simulink model "fractional_6"  (Simulink 7.4)
settings: Solver=ode45  StartTime=0.0  StopTime=1e-4  FixedStep=.01/(fr*N/M)  MaxStep=1/(3*fr*N)  RelTol=1e-7  AbsTol=1e-3
PreLoadFcn:
  | fr=10e6,fi=99e6,sen=10e6,N=10,M=.015
StartFcn:
  | tic
StopFcn:
  | trun=toc
undefined symbols (not defined in the file or in its folder): dBW, Hz, M, N, One, sen, sided
libraries: powerlib x11, dspstat3 x4, dsparch4 x3, simulink x3, simulink_extras x2, dspsnks4 x2, commsynccomp2 x1
settings Model: Creator=d benson  LastModifiedBy=Dick  ModifiedHistory=digital phase correction added, Benson, Fall 2001  BufferReuse=off
settings DataIOCC: LimitDataPoints=off  SaveOutput=off  SaveTime=off  SignalLoggingName=sigsOut
settings OptimizationCC: BlockReduction=off  BooleanDataType=off  InlineInvariantSignals=on  OptimizeBlockIOStorage=off  BufferReuse=off  ExpressionFolding=off  LocalBlockOutputs=off  InitFltsAndDblsToZero=on
settings DebuggingCC: SaveWithParameterizedLinksMsg=none  SignalResolutionControl=TryResolveAllWithWarning  SolverPrmCheckMsg=none  MultiTaskDSMMsg=warning  MultiTaskCondExecSysMsg=none  StrictBusMsg=None
settings HardwareCC: TargetUnknown=on
settings RTWCC: IncludeERTFirstTime=on
settings GRTTargetCC: TargetFcnLib=ansi_tfl_tmw.mat

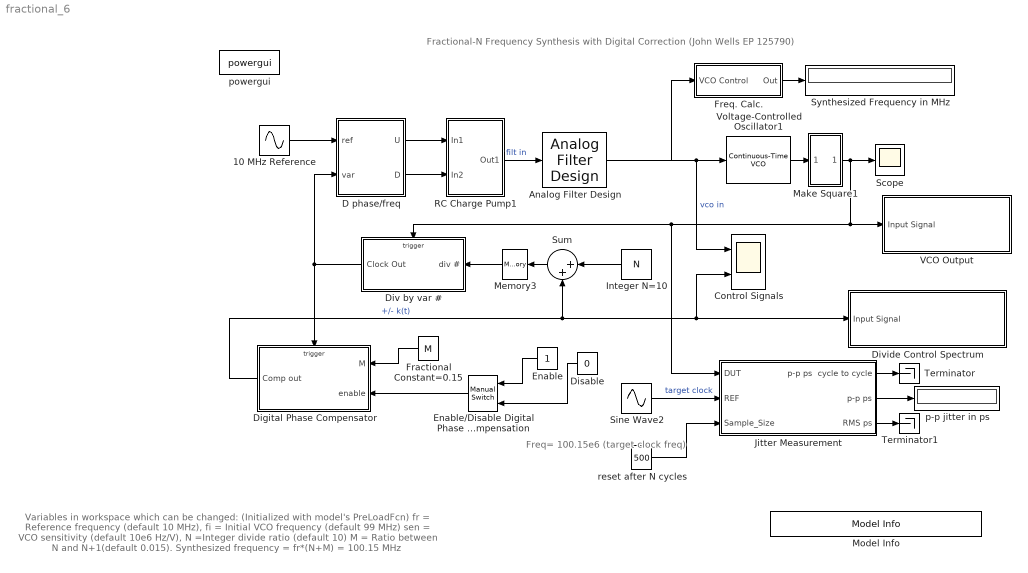
== system fractional_6 ==
  note: Fractional-N Frequency Synthesis with Digital Correction (John Wells EP 125790)
  note: Variables in workspace which can be changed: (Initialized with model's PreLoadFcn)
      | fr = Reference frequency (default 10  MHz),        fi = Initial VCO frequency (default 99 MHz)
      | sen = VCO sensitivity (default 10e6 Hz/V),         N =Integer divide ratio (default 10)
      | M = Ratio between N and N+1(default 0.015).     Synthesized frequency = fr*(N+M) = 100.15 MHz
  note: Freq= 100.15e6 (target clock freq)
  10 MHz Reference : Sin  Amplitude=1  Bias=0  Frequency=2*pi*fr  Phase=0  Samples=10  SampleTime=0  Offset=0
  Analog Filter Design : dsparch4/Analog Filter Design  method=Elliptic  filttype=Lowpass  N=6  Wlo=2*pi*1e6  Whi=80  Rp=2  Rs=80
  Control Signals : Scope  NumInputPorts=2
      settings: TimeRange=0.0001  YMin=0~-7.5  YMax=0.2~7.5  Decimation=51
  "D phase/freq " : Subsystem
  Digital Phase Compensator : Subsystem  TreatAsAtomicUnit=on
  Disable : Constant  Value=0  OutDataType=sfix(16)  OutScaling=2^0
  Div by var # : Subsystem  TreatAsAtomicUnit=on
  Divide Control Spectrum : Subsystem  Description=Spectrum Analyzer  mask{BW=40e6}
      mask prompts: BW "Bandwidth"
      mask Display: fprintf('Baseband Spectrum Analyzer \n  BW=%7.2f MHz', BW/1e6)
  Enable : Constant  OutDataType=sfix(16)  OutScaling=2^0
  Enable/Disable Digital Phase Compensation : simulink/Signal Routing/Manual Switch  SystemSampleTime=-1  sw=1  action=0  varsize=off
  Fractional Constant=0.15 : Constant  Value=M  OutDataType=sfix(16)  OutScaling=2^0
  Freq. Calc. : Subsystem
  Integer N=10 : Constant  Value=N  OutDataType=sfix(16)  OutScaling=2^0
  "Jitter Measurement " : Subsystem
  Make Square1 : Subsystem
      mask Type: Make Square
      mask Description:
      | For input +ve values output is 1
      | For input -ve values output is 0
      mask Display: plot(0,0,100,100,[90,70,70,50,50,30,30,10,10],[20,20,40,40,20,20,40,40,20],[90,87,84,80,76,73,70,67,63,60,57,53,50,47,44,40,36,33,30,27,23,20,17,13,10],[70,65,63,62,63,65,70,75,77,78,77,75,70,65,63,62,63,65,70,75,77,78,77,75,70])
  Memory3 : Memory
  Model Info : simulink/Model-Wide Utilities/Model Info  SystemSampleTime=-1  InitialBlockCM=none  BlockCM=none  Frame=on  DisplayStringWithTags=Copywrite 2005-2010 The MathWorks, Inc.  HorizontalTextAlignment=Center  LeftAlignmentValue=0.5  SourceBlockDiagram=fractional_6  TagMaxNumber=20
  RC Charge Pump1 : Subsystem
  Scope : Scope
      settings: TimeRange=9.98502246630055e-009  YMin=-0.1  YMax=1.1
  Sine Wave2 : Sin  Amplitude=1  Bias=0  Frequency=2*pi*(100.15e6)  Phase=pi/2  Samples=10  SampleTime=0  Offset=0
  Sum : Sum  Inputs=|++  OutDataType=sfix(16)  OutScaling=2^0  SaturateOnIntegerOverflow=on  InputSameDT=on  OutDataTypeStr=Inherit: Same as first input
  "Synthesized Frequency in MHz " : Display
      settings: Decimation=401
  Terminator : Terminator
  Terminator1 : Terminator
  VCO Output : Subsystem  Description=Spectrum Analyzer  mask{BW=4e6, Fc=100.15e6}
      mask prompts: BW "Bandwidth"; Fc "Center Freq"
      mask Display: fprintf('Spectrum Analyzer \n Fc=%7.2f MHz \n BW=%7.2f MHz',Fc/1e6,BW/1e6)
  Voltage-Controlled Oscillator1 : commsynccomp2/Continuous-Time VCO  SystemSampleTime=-1  Ac=1  Fc=fi  Kc=sen  Ph=pi/8
  p-p jitter in ps : Display
  powergui : powerlib/powergui  SystemSampleTime=-1  SimulationMode=Continuous  SampleTime=0  frequency=60  SPID=off  DisableSnubberDevices=off  DisableRonSwitches=off  DisableVfSwitches=off  SwTol=0  Interpol=off  frequencyindice=0  echomessages=off  HookPort=off  DisplayEquations=off  FunctionMessages=off  EnableUseOfTLC=off  x0status=blocks  RestoreLinks=warning  Frange=[0:2:500]  Ylog=off  Xlog=on  ShowGrid=off  save=off  variable=ZData  ZoomFFT=on  StartTime=0.0  cycles=1  DisplayStyle=1  fundamental=60  FreqAxis=off  MaxFrequency=1000  frequencyindicesteady=1  RmsSteady=1  display=off  Ts=0  methode=off
  reset after N cycles : Constant  Value=500  VectorParams1D=off  OutDataType=sfix(16)  OutScaling=2^0
  wires:
  Voltage-Controlled Oscillator1/1 -> Make Square1/1(In1)
  Make Square1/1(Out1) -> Scope/1, VCO Output/1(Input Signal), Div by var #/Trigger, "Jitter Measurement "/1(DUT)
  10 MHz Reference/1 -> "D phase/freq "/1(ref)
  Div by var #/1(Clock Out) -> "D phase/freq "/2(var), Digital Phase Compensator/Trigger
  Sum/1 -> Memory3/1
  Integer N=10/1 -> Sum/1
  Freq. Calc./1(Out) -> "Synthesized Frequency in MHz "/1
  Analog Filter Design/1 -> Control Signals/1, Freq. Calc./1(VCO Control), Voltage-Controlled Oscillator1/1  "vco in"
  "D phase/freq "/1(U) -> RC Charge Pump1/1(In1)
  "D phase/freq "/2(D) -> RC Charge Pump1/2(In2)
  RC Charge Pump1/1(Out1) -> Analog Filter Design/1  "filt in"
  Digital Phase Compensator/1(Comp out) -> Sum/2, Control Signals/2, Divide Control Spectrum/1(Input Signal)  "+/- k(t)"
  Fractional Constant=0.15/1 -> Digital Phase Compensator/1(M)
  Enable/Disable Digital Phase Compensation/1 -> Digital Phase Compensator/2(enable)
  Enable/1 -> Enable/Disable Digital Phase Compensation/1
  Disable/1 -> Enable/Disable Digital Phase Compensation/2
  Sine Wave2/1 -> "Jitter Measurement "/2(REF)  "target clock"
  "Jitter Measurement "/2(p-p ps) -> p-p jitter in ps/1
  reset after N cycles/1 -> "Jitter Measurement "/3(Sample_Size)
  Memory3/1 -> Div by var #/1(div #)
  "Jitter Measurement "/1(p-p ps  cycle to cycle) -> Terminator/1
  "Jitter Measurement "/3(RMS ps) -> Terminator1/1

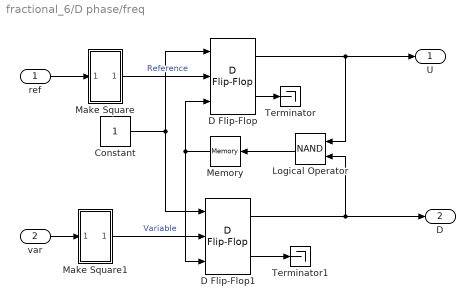
== system fractional_6/D phase/freq  ==
  ref : Inport  OutDataType=sfix(16)  OutScaling=2^0
  var : Inport  Port=2  OutDataType=sfix(16)  OutScaling=2^0
  Constant : Constant  OutDataType=sfix(16)  OutScaling=2^0
  D Flip-Flop : simulink_extras/Flip Flops/D Flip-Flop  SystemSampleTime=-1
  D Flip-Flop1 : simulink_extras/Flip Flops/D Flip-Flop  SystemSampleTime=-1
  Logical Operator : Logic  Operator=NAND
  Make Square : Subsystem
      mask Type: Make Square
      mask Description:
      | For input +ve values output is 1
      | For input -ve values output is 0
      mask Display: plot(0,0,100,100,[90,70,70,50,50,30,30,10,10],[20,20,40,40,20,20,40,40,20],[90,87,84,80,76,73,70,67,63,60,57,53,50,47,44,40,36,33,30,27,23,20,17,13,10],[70,65,63,62,63,65,70,75,77,78,77,75,70,65,63,62,63,65,70,75,77,78,77,75,70])
  Make Square1 : Subsystem
      mask Type: Make Square
      mask Description:
      | For input +ve values output is 1
      | For input -ve values output is 0
      mask Display: plot(0,0,100,100,[90,70,70,50,50,30,30,10,10],[20,20,40,40,20,20,40,40,20],[90,87,84,80,76,73,70,67,63,60,57,53,50,47,44,40,36,33,30,27,23,20,17,13,10],[70,65,63,62,63,65,70,75,77,78,77,75,70,65,63,62,63,65,70,75,77,78,77,75,70])
  Memory : Memory
  Terminator : Terminator
  Terminator1 : Terminator
  U : Outport  OutDataType=sfix(16)  OutScaling=2^0
  D : Outport  Port=2  OutDataType=sfix(16)  OutScaling=2^0
  wires:
  D Flip-Flop1/1 -> Logical Operator/2, D/1
  D Flip-Flop/1 -> Logical Operator/1, U/1
  Memory/1 -> D Flip-Flop1/3, D Flip-Flop/3
  Make Square1/1(Out1) -> D Flip-Flop1/2  "Variable"
  Make Square/1(Out1) -> D Flip-Flop/2  "Reference"
  Constant/1 -> D Flip-Flop1/1, D Flip-Flop/1
  var/1 -> Make Square1/1(In1)
  ref/1 -> Make Square/1(In1)
  Logical Operator/1 -> Memory/1
  D Flip-Flop1/2 -> Terminator1/1
  D Flip-Flop/2 -> Terminator/1

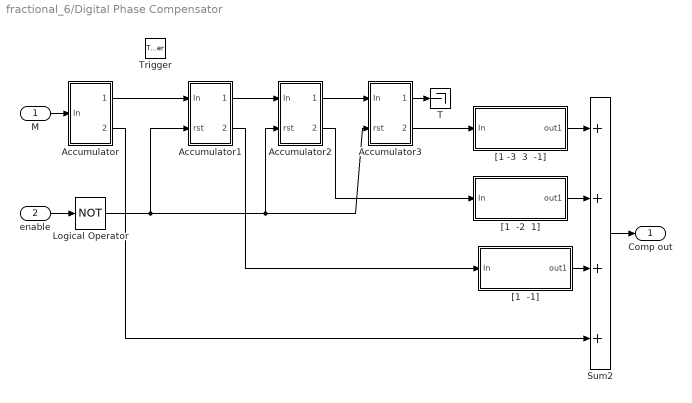
== system fractional_6/Digital Phase Compensator ==
  M : Inport  OutDataType=sfix(16)  OutScaling=2^0
  enable : Inport  Port=2  OutDataType=sfix(16)  OutScaling=2^0
  Trigger : TriggerPort
  Accumulator : Subsystem
  Accumulator1 : Subsystem
  Accumulator2 : Subsystem
  Accumulator3 : Subsystem
  Logical Operator : Logic  Operator=NOT
  Sum2 : Sum  Inputs=++++  OutDataType=sfix(16)  OutScaling=2^0  SaturateOnIntegerOverflow=on  InputSameDT=on  OutDataTypeStr=Inherit: Same as first input
  T : Terminator
  "[1  -1] " : Subsystem  TreatAsAtomicUnit=on
  "[1  -2  1]" : Subsystem  TreatAsAtomicUnit=on
  "[1 -3  3  -1]" : Subsystem  TreatAsAtomicUnit=on
  Comp out : Outport  OutDataType=sfix(16)  OutScaling=2^0
  wires:
  M/1 -> Accumulator/1(In)
  Accumulator1/1(State) -> Accumulator2/1(In)
  Accumulator2/1(State) -> Accumulator3/1(In)
  Accumulator1/2(Carry) -> "[1  -1] "/1(In)
  Accumulator2/2(Carry) -> "[1  -2  1]"/1(In)
  Accumulator3/2(Carry) -> "[1 -3  3  -1]"/1(In)
  Accumulator3/1(State) -> T/1
  Accumulator/1(State) -> Accumulator1/1(In)
  Sum2/1 -> Comp out/1
  "[1 -3  3  -1]"/1(out1) -> Sum2/1
  "[1  -2  1]"/1(out1) -> Sum2/2
  "[1  -1] "/1(out1) -> Sum2/3
  Accumulator/2(Carry) -> Sum2/4
  enable/1 -> Logical Operator/1
  Logical Operator/1 -> Accumulator1/2(rst), Accumulator2/2(rst), Accumulator3/2(rst)

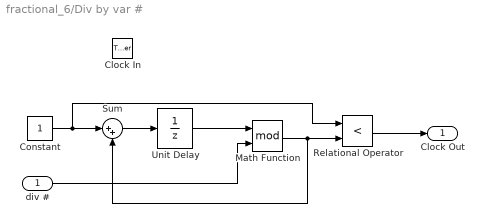
== system fractional_6/Div by var # ==
  div # : Inport  OutDataType=sfix(16)  OutScaling=2^0
  Clock In : TriggerPort
  Constant : Constant  OutDataType=sfix(16)  OutScaling=2^0
  Math Function : Math  Operator=mod  OutDataType=sfix(16)  OutScaling=2^0  SaturateOnIntegerOverflow=on
  Relational Operator : RelationalOperator  Operator=<  InputSameDT=on
  Sum : Sum  Inputs=|++  OutDataType=sfix(16)  OutScaling=2^0  SaturateOnIntegerOverflow=on  InputSameDT=on  OutDataTypeStr=Inherit: Same as first input
  Unit Delay : UnitDelay  SampleTime=-1
  Clock Out : Outport  OutDataType=sfix(16)  OutScaling=2^0
  wires:
  Constant/1 -> Sum/1, Relational Operator/1
  Sum/1 -> Unit Delay/1
  Unit Delay/1 -> Math Function/1
  div #/1 -> Math Function/2
  Math Function/1 -> Sum/2, Relational Operator/2
  Relational Operator/1 -> Clock Out/1

== system fractional_6/Divide Control Spectrum ==
  Input Signal : Inport  OutDataType=sfix(16)  OutScaling=2^0
  Spectrum Scope : dspsnks4/Spectrum Scope  DialogController=dspdialog.SpectrumScope  DialogControllerArgs=DataTag0  SystemSampleTime=-1  ScopeProperties=on  Domain=Frequency  HorizSpan=1  UseBuffer=on  BufferSize=256  Overlap=0  inpFftLenInherit=off  FFTlength=128  numAvg=1  DisplayProperties=off  AxisGrid=on  Memory=off  FrameNumber=on  AxisLegend=off  AxisZoom=off  OpenScopeAtSimStart=on  OpenScopeImmediately=off  FigPos=[386 37 333 196]  AxisProperties=off  XUnits=Hertz  XRange=One-sided ([0...Fs/2])  XDisplay=0  InheritXIncr=on  XIncr=1.0  XLabel=Samples  XLimit=Auto  YUnits=dBW  XMax=1  XMin=0  YLabel=dBW/Hz  LineProperties=off  wintypeSpecScope=Hann  RsSpecScope=50  betaSpecScope=5  winsampSpecScope=Periodic  XAxisParamsVer=6.9
      settings: YMin=-100  YMax=0
  anti alias : dsparch4/Analog Filter Design  method=Elliptic  filttype=Lowpass  N=8  Wlo=BW*2*pi  Whi=80  Rp=0.11  Rs=100
  sampler : ZeroOrderHold  SampleTime=1/(2.56*BW)
  wires:
  sampler/1 -> Spectrum Scope/1
  anti alias/1 -> sampler/1
  Input Signal/1 -> anti alias/1

== system fractional_6/Freq. Calc. ==
  VCO Control : Inport  OutDataType=sfix(16)  OutScaling=2^0
  F : Constant  Value=fi  OutDataType=sfix(16)  OutScaling=2^0
  Gain1 : Gain  Gain=1e-6  ParameterDataType=sfix(16)  ParameterScaling=2^0  OutDataType=sfix(16)  OutScaling=2^0  SaturateOnIntegerOverflow=on  OutDataTypeStr=Inherit: Same as input  ParamDataTypeStr=Inherit: Same as input
  Gain3 : Gain  Gain=sen  ParameterDataType=sfix(16)  ParameterScaling=2^0  OutDataType=sfix(16)  OutScaling=2^0  SaturateOnIntegerOverflow=on  OutDataTypeStr=Inherit: Same as input  ParamDataTypeStr=Inherit: Same as input
  Sum1 : Sum  Inputs=|++  OutDataType=sfix(16)  OutScaling=2^0  SaturateOnIntegerOverflow=on  InputSameDT=on  OutDataTypeStr=Inherit: Same as first input
  Out : Outport  OutDataType=sfix(16)  OutScaling=2^0
  wires:
  Sum1/1 -> Gain1/1
  F/1 -> Sum1/2
  Gain3/1 -> Sum1/1
  VCO Control/1 -> Gain3/1
  Gain1/1 -> Out/1

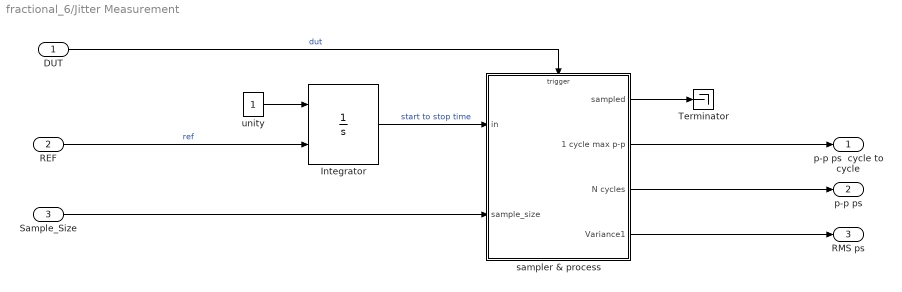
== system fractional_6/Jitter Measurement  ==
  DUT : Inport  OutDataType=sfix(16)  OutScaling=2^0
  REF : Inport  Port=2  OutDataType=sfix(16)  OutScaling=2^0
  Sample_Size : Inport  Port=3  OutDataType=sfix(16)  OutScaling=2^0
  Integrator : Integrator  ExternalReset=rising
  Terminator : Terminator
  sampler & process : Subsystem  TreatAsAtomicUnit=on
  unity : Constant  OutDataTypeMode=double  OutDataType=sfix(16)  OutScaling=2^0  OutDataTypeStr=double
  p-p ps  cycle to cycle : Outport  OutDataType=sfix(16)  OutScaling=2^0
  p-p ps : Outport  Port=2  OutDataType=sfix(16)  OutScaling=2^0
  RMS ps : Outport  Port=3  OutDataType=sfix(16)  OutScaling=2^0
  wires:
  DUT/1 -> sampler & process/Trigger  "dut"
  REF/1 -> Integrator/2  "ref"
  Integrator/1 -> sampler & process/1(in)  "start to stop time"
  Sample_Size/1 -> sampler & process/2(sample_size)
  sampler & process/3(N cycles) -> p-p ps/1
  sampler & process/4(Variance1) -> RMS ps/1
  unity/1 -> Integrator/1
  sampler & process/2(1 cycle max p-p) -> p-p ps  cycle to cycle/1
  sampler & process/1(sampled) -> Terminator/1

== system fractional_6/Make Square1 ==
  In1 : Inport  OutDataType=sfix(16)  OutScaling=2^0
  Constant : Constant  Value=0  OutDataType=sfix(16)  OutScaling=2^0
  Relational Operator : RelationalOperator  Operator=>  InputSameDT=on
  Out1 : Outport  OutDataType=sfix(16)  OutScaling=2^0
  wires:
  In1/1 -> Relational Operator/1
  Constant/1 -> Relational Operator/2
  Relational Operator/1 -> Out1/1

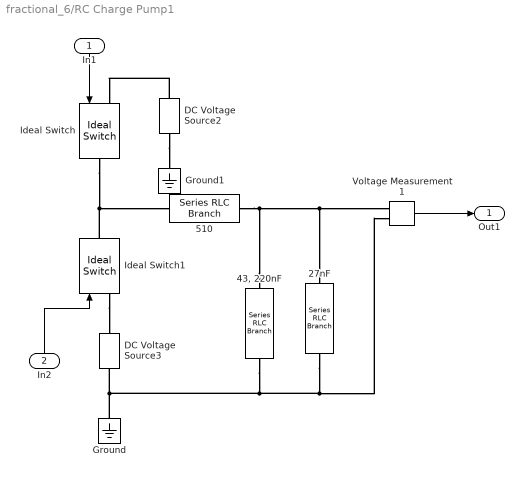
== system fractional_6/RC Charge Pump1 ==
  In1 : Inport  OutDataType=sfix(16)  OutScaling=2^0
  In2 : Inport  Port=2  OutDataType=sfix(16)  OutScaling=2^0
  27nF : powerlib/Elements/Series RLC Branch  DialogController=POWERSYS.PowerSysDialog  PhysicalDomain=powersysdomain  SubClassName=unknown  LeftPortType=p1  RightPortType=p1  LConnTagsString=__new0  RConnTagsString=__new0  BranchType=C  Resistance=3900  Inductance=1e-3  SetiL0=off  InitialCurrent=0  Capacitance=27e-9  Setx0=off  InitialVoltage=0  Measurements=None
  "43, 220nF" : powerlib/Elements/Series RLC Branch  DialogController=POWERSYS.PowerSysDialog  PhysicalDomain=powersysdomain  SubClassName=unknown  LeftPortType=p1  RightPortType=p1  LConnTagsString=__new0  RConnTagsString=__new0  BranchType=RC  Resistance=43  Inductance=1e-3  SetiL0=off  InitialCurrent=0  Capacitance=220e-9  Setx0=off  InitialVoltage=0  Measurements=None
  510 : powerlib/Elements/Series RLC Branch  DialogController=POWERSYS.PowerSysDialog  PhysicalDomain=powersysdomain  SubClassName=unknown  LeftPortType=p1  RightPortType=p1  LConnTagsString=__new0  RConnTagsString=__new0  BranchType=R  Resistance=510  Inductance=1e-3  SetiL0=off  InitialCurrent=0  Capacitance=1e-6  Setx0=off  InitialVoltage=0  Measurements=None
  DC Voltage Source2 : powerlib/Electrical Sources/DC Voltage Source  DialogController=POWERSYS.PowerSysDialog  SystemSampleTime=-1  Amplitude=5  Measurements=None
  DC Voltage Source3 : powerlib/Electrical Sources/DC Voltage Source  DialogController=POWERSYS.PowerSysDialog  SystemSampleTime=-1  Amplitude=-5  Measurements=None
  Ground : powerlib/Elements/Ground  DialogController=POWERSYS.PowerSysDialog  PhysicalDomain=powersysdomain  SubClassName=unknown  LeftPortType=p1  RightPortType=p1  LConnTagsString=a
  Ground1 : powerlib/Elements/Ground  DialogController=POWERSYS.PowerSysDialog  PhysicalDomain=powersysdomain  SubClassName=unknown  LeftPortType=p1  RightPortType=p1  LConnTagsString=a
  Ideal Switch : powerlib/Power Electronics/Ideal Switch  DialogController=POWERSYS.PowerSysDialog  SystemSampleTime=-1  Ron=10  Lon=0  IC=0  Rs=inf  Cs=inf  Measurements=off
  Ideal Switch1 : powerlib/Power Electronics/Ideal Switch  DialogController=POWERSYS.PowerSysDialog  SystemSampleTime=-1  Ron=10  Lon=0  IC=0  Rs=inf  Cs=inf  Measurements=off
  Voltage Measurement1 : powerlib/Measurements/Voltage Measurement  DialogController=POWERSYS.PowerSysDialog  SystemSampleTime=-1  PhasorSimulation=off  OutputType=Complex  PSBequivalent=0
  Out1 : Outport  OutDataType=sfix(16)  OutScaling=2^0
  wires:
  In2/1 -> Ideal Switch1/1
  Voltage Measurement1/1 -> Out1/1
  In1/1 -> Ideal Switch/1
  connections:
  Voltage Measurement1/LConn2 -- 27nF/RConn1 -- "43, 220nF"/RConn1 -- Ground/LConn1 -- DC Voltage Source3/LConn1
  "43, 220nF"/LConn1 -- Voltage Measurement1/LConn1 -- 27nF/LConn1 -- 510/RConn1
  Ideal Switch1/RConn1 -- Ideal Switch/RConn1 -- 510/LConn1
  DC Voltage Source2/LConn1 -- Ground1/LConn1
  Ideal Switch1/LConn1 -- DC Voltage Source3/RConn1
  DC Voltage Source2/RConn1 -- Ideal Switch/LConn1

== system fractional_6/VCO Output ==
  Input Signal : Inport  OutDataType=sfix(16)  OutScaling=2^0
  Sine Wave1 : Sin  Amplitude=2*sqrt(2)  Bias=0  Frequency=2*pi*(Fc-BW/2)  Phase=-pi/2  Samples=10  SampleTime=0  Offset=0
  Spectrum Scope : dspsnks4/Spectrum Scope  DialogController=dspdialog.SpectrumScope  DialogControllerArgs=DataTag5  SystemSampleTime=-1  ScopeProperties=on  Domain=Frequency  HorizSpan=1  UseBuffer=on  BufferSize=512  Overlap=512-128  inpFftLenInherit=off  FFTlength=128  numAvg=1  DisplayProperties=off  AxisGrid=on  Memory=off  FrameNumber=on  AxisLegend=off  AxisZoom=off  OpenScopeAtSimStart=on  OpenScopeImmediately=off  FigPos=[48 37 329 194]  AxisProperties=off  XUnits=Hertz  XRange=One-sided ([0...Fs/2])  XDisplay=0  InheritXIncr=on  XIncr=1.0  XLabel=Samples  XLimit=Auto  YUnits=dBW  XMax=1  XMin=0  YLabel=dBW  LineProperties=off  wintypeSpecScope=Hann  RsSpecScope=50  betaSpecScope=5  winsampSpecScope=Periodic  XAxisParamsVer=6.9
      settings: YMin=-100  YMax=20
  anti alias : dsparch4/Analog Filter Design  method=Elliptic  filttype=Lowpass  N=9  Wlo=BW*2*pi  Whi=80  Rp=2  Rs=80
  down convert : Product  OutDataType=sfix(16)  OutScaling=2^0  SaturateOnIntegerOverflow=on  InputSameDT=on  OutDataTypeStr=Inherit: Same as first input
  sampler : ZeroOrderHold  SampleTime=1/(2.56*BW)
  wires:
  Sine Wave1/1 -> down convert/1
  sampler/1 -> Spectrum Scope/1
  anti alias/1 -> sampler/1
  down convert/1 -> anti alias/1
  Input Signal/1 -> down convert/2

== system fractional_6/D phase/freq /Make Square ==
  In1 : Inport  OutDataType=sfix(16)  OutScaling=2^0
  Constant : Constant  Value=0  OutDataType=sfix(16)  OutScaling=2^0
  Relational Operator : RelationalOperator  Operator=>  InputSameDT=on
  Out1 : Outport  OutDataType=sfix(16)  OutScaling=2^0
  wires:
  In1/1 -> Relational Operator/1
  Constant/1 -> Relational Operator/2
  Relational Operator/1 -> Out1/1

== system fractional_6/D phase/freq /Make Square1 ==
  In1 : Inport  OutDataType=sfix(16)  OutScaling=2^0
  Constant : Constant  Value=0  OutDataType=sfix(16)  OutScaling=2^0
  Relational Operator : RelationalOperator  Operator=>  InputSameDT=on
  Out1 : Outport  OutDataType=sfix(16)  OutScaling=2^0
  wires:
  In1/1 -> Relational Operator/1
  Constant/1 -> Relational Operator/2
  Relational Operator/1 -> Out1/1

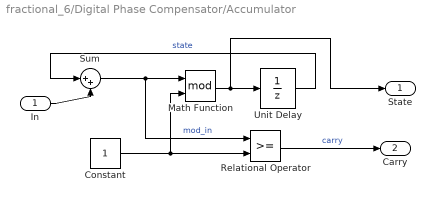
== system fractional_6/Digital Phase Compensator/Accumulator ==
  In : Inport  OutDataType=sfix(16)  OutScaling=2^0
  Constant : Constant  OutDataType=sfix(16)  OutScaling=2^0
  Math Function : Math  Operator=mod  OutDataType=sfix(16)  OutScaling=2^0  SaturateOnIntegerOverflow=on
  Relational Operator : RelationalOperator  InputSameDT=on
  Sum : Sum  Inputs=|++  OutDataType=sfix(16)  OutScaling=2^0  SaturateOnIntegerOverflow=on  InputSameDT=on  OutDataTypeStr=Inherit: Same as first input
  Unit Delay : UnitDelay  SampleTime=-1
  State : Outport  OutDataType=sfix(16)  OutScaling=2^0
  Carry : Outport  Port=2  OutDataType=sfix(16)  OutScaling=2^0
  wires:
  In/1 -> Sum/2
  Unit Delay/1 -> Sum/1  "state"
  Sum/1 -> Math Function/1, Relational Operator/1  "mod_in"
  Math Function/1 -> State/1, Unit Delay/1
  Constant/1 -> Math Function/2, Relational Operator/2
  Relational Operator/1 -> Carry/1  "carry"

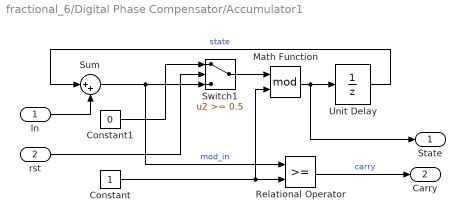
== system fractional_6/Digital Phase Compensator/Accumulator1 ==
  In : Inport  OutDataType=sfix(16)  OutScaling=2^0
  rst : Inport  Port=2  OutDataType=sfix(16)  OutScaling=2^0
  Constant : Constant  OutDataType=sfix(16)  OutScaling=2^0
  Constant1 : Constant  Value=0  OutDataType=sfix(16)  OutScaling=2^0
  Math Function : Math  Operator=mod  OutDataType=sfix(16)  OutScaling=2^0  SaturateOnIntegerOverflow=on
  Relational Operator : RelationalOperator  InputSameDT=on
  Sum : Sum  Inputs=|++  OutDataType=sfix(16)  OutScaling=2^0  SaturateOnIntegerOverflow=on  InputSameDT=on  OutDataTypeStr=Inherit: Same as first input
  Switch1 : Switch  Threshold=0.5  SaturateOnIntegerOverflow=on  InputSameDT=on
  Unit Delay : UnitDelay  SampleTime=-1
  State : Outport  OutDataType=sfix(16)  OutScaling=2^0
  Carry : Outport  Port=2  OutDataType=sfix(16)  OutScaling=2^0
  wires:
  Relational Operator/1 -> Carry/1  "carry"
  Constant/1 -> Relational Operator/2, Math Function/2
  Math Function/1 -> State/1, Unit Delay/1
  Sum/1 -> Relational Operator/1, Switch1/3  "mod_in"
  Unit Delay/1 -> Sum/1  "state"
  In/1 -> Sum/2
  Switch1/1 -> Math Function/1
  Constant1/1 -> Switch1/1
  rst/1 -> Switch1/2

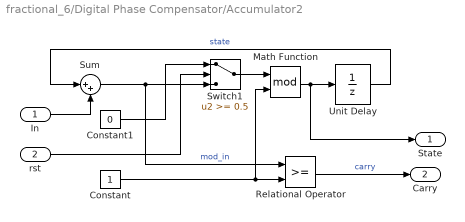
== system fractional_6/Digital Phase Compensator/Accumulator2 ==
  In : Inport  OutDataType=sfix(16)  OutScaling=2^0
  rst : Inport  Port=2  OutDataType=sfix(16)  OutScaling=2^0
  Constant : Constant  OutDataType=sfix(16)  OutScaling=2^0
  Constant1 : Constant  Value=0  OutDataType=sfix(16)  OutScaling=2^0
  Math Function : Math  Operator=mod  OutDataType=sfix(16)  OutScaling=2^0  SaturateOnIntegerOverflow=on
  Relational Operator : RelationalOperator  InputSameDT=on
  Sum : Sum  Inputs=|++  OutDataType=sfix(16)  OutScaling=2^0  SaturateOnIntegerOverflow=on  InputSameDT=on  OutDataTypeStr=Inherit: Same as first input
  Switch1 : Switch  Threshold=0.5  SaturateOnIntegerOverflow=on  InputSameDT=on
  Unit Delay : UnitDelay  SampleTime=-1
  State : Outport  OutDataType=sfix(16)  OutScaling=2^0
  Carry : Outport  Port=2  OutDataType=sfix(16)  OutScaling=2^0
  wires:
  rst/1 -> Switch1/2
  Constant1/1 -> Switch1/1
  Switch1/1 -> Math Function/1
  In/1 -> Sum/2
  Unit Delay/1 -> Sum/1  "state"
  Sum/1 -> Switch1/3, Relational Operator/1  "mod_in"
  Math Function/1 -> Unit Delay/1, State/1
  Constant/1 -> Math Function/2, Relational Operator/2
  Relational Operator/1 -> Carry/1  "carry"

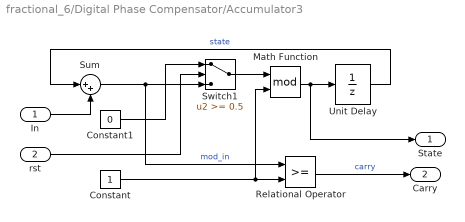
== system fractional_6/Digital Phase Compensator/Accumulator3 ==
  In : Inport  OutDataType=sfix(16)  OutScaling=2^0
  rst : Inport  Port=2  OutDataType=sfix(16)  OutScaling=2^0
  Constant : Constant  OutDataType=sfix(16)  OutScaling=2^0
  Constant1 : Constant  Value=0  OutDataType=sfix(16)  OutScaling=2^0
  Math Function : Math  Operator=mod  OutDataType=sfix(16)  OutScaling=2^0  SaturateOnIntegerOverflow=on
  Relational Operator : RelationalOperator  InputSameDT=on
  Sum : Sum  Inputs=|++  OutDataType=sfix(16)  OutScaling=2^0  SaturateOnIntegerOverflow=on  InputSameDT=on  OutDataTypeStr=Inherit: Same as first input
  Switch1 : Switch  Threshold=0.5  SaturateOnIntegerOverflow=on  InputSameDT=on
  Unit Delay : UnitDelay  SampleTime=-1
  State : Outport  OutDataType=sfix(16)  OutScaling=2^0
  Carry : Outport  Port=2  OutDataType=sfix(16)  OutScaling=2^0
  wires:
  Relational Operator/1 -> Carry/1  "carry"
  Constant/1 -> Relational Operator/2, Math Function/2
  Math Function/1 -> State/1, Unit Delay/1
  Sum/1 -> Relational Operator/1, Switch1/3  "mod_in"
  Unit Delay/1 -> Sum/1  "state"
  In/1 -> Sum/2
  Switch1/1 -> Math Function/1
  Constant1/1 -> Switch1/1
  rst/1 -> Switch1/2

== system fractional_6/Digital Phase Compensator/[1  -1]  ==
  In : Inport  OutDataType=sfix(16)  OutScaling=2^0
  Sum : Sum  Inputs=|+-  OutDataType=sfix(16)  OutScaling=2^0  SaturateOnIntegerOverflow=on  InputSameDT=on  OutDataTypeStr=Inherit: Same as first input
  Unit Delay : UnitDelay  SampleTime=-1
  out1 : Outport  OutDataType=sfix(16)  OutScaling=2^0
  wires:
  In/1 -> Unit Delay/1, Sum/1
  Unit Delay/1 -> Sum/2
  Sum/1 -> out1/1

== system fractional_6/Digital Phase Compensator/[1  -2  1] ==
  In : Inport  OutDataType=sfix(16)  OutScaling=2^0
  Gain : Gain  Gain=-2  ParameterDataType=sfix(16)  ParameterScaling=2^0  OutDataType=sfix(16)  OutScaling=2^0  SaturateOnIntegerOverflow=on  OutDataTypeStr=Inherit: Same as input  ParamDataTypeStr=Inherit: Same as input
  Sum : Sum  Inputs=+++  OutDataType=sfix(16)  OutScaling=2^0  SaturateOnIntegerOverflow=on  InputSameDT=on  OutDataTypeStr=Inherit: Same as first input
  Unit Delay : UnitDelay  SampleTime=-1
  Unit Delay1 : UnitDelay  SampleTime=-1
  out1 : Outport  OutDataType=sfix(16)  OutScaling=2^0
  wires:
  Gain/1 -> Sum/2
  Unit Delay/1 -> Gain/1, Unit Delay1/1
  In/1 -> Unit Delay/1, Sum/1
  Unit Delay1/1 -> Sum/3
  Sum/1 -> out1/1

== system fractional_6/Digital Phase Compensator/[1 -3  3  -1] ==
  In : Inport  OutDataType=sfix(16)  OutScaling=2^0
  Gain : Gain  Gain=-3  ParameterDataType=sfix(16)  ParameterScaling=2^0  OutDataType=sfix(16)  OutScaling=2^0  SaturateOnIntegerOverflow=on  OutDataTypeStr=Inherit: Same as input  ParamDataTypeStr=Inherit: Same as input
  Gain1 : Gain  Gain=3  ParameterDataType=sfix(16)  ParameterScaling=2^0  OutDataType=sfix(16)  OutScaling=2^0  SaturateOnIntegerOverflow=on  OutDataTypeStr=Inherit: Same as input  ParamDataTypeStr=Inherit: Same as input
  Sum : Sum  Inputs=+++-  OutDataType=sfix(16)  OutScaling=2^0  SaturateOnIntegerOverflow=on  InputSameDT=on  OutDataTypeStr=Inherit: Same as first input
  Unit Delay : UnitDelay  SampleTime=-1
  Unit Delay1 : UnitDelay  SampleTime=-1
  Unit Delay2 : UnitDelay  SampleTime=-1
  out1 : Outport  OutDataType=sfix(16)  OutScaling=2^0
  wires:
  In/1 -> Sum/1, Unit Delay/1
  Unit Delay/1 -> Unit Delay1/1, Gain/1
  Unit Delay1/1 -> Gain1/1, Unit Delay2/1
  Gain/1 -> Sum/2
  Gain1/1 -> Sum/3
  Unit Delay2/1 -> Sum/4
  Sum/1 -> out1/1

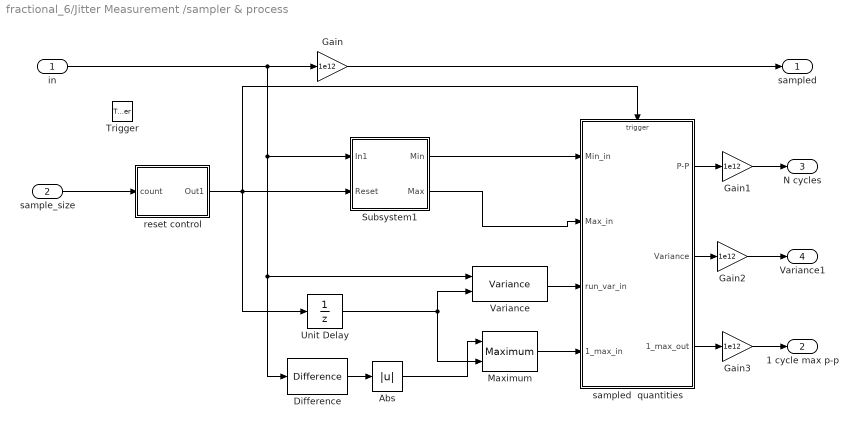
== system fractional_6/Jitter Measurement /sampler & process ==
  in : Inport  OutDataType=sfix(16)  OutScaling=2^0
  sample_size : Inport  Port=2  OutDataType=sfix(16)  OutScaling=2^0
  Trigger : TriggerPort
  Abs : Abs
  Difference : simulink/Discrete/Difference  SystemSampleTime=-1  ICPrevInput=0.0  OutMin=[]  OutMax=[]  OutDataType=sfix(16)  OutScaling=2^-10  DoSatur=off
  Gain{,1..3} (4 alike) : Gain  Gain=1e12  ParameterDataType=sfix(16)  ParameterScaling=2^0  OutDataType=sfix(16)  OutScaling=2^0
  Maximum : dspstat3/Maximum  DialogController=dspDDGCreate  DialogControllerArgs=DataTag1  fcn=Running  reset=Rising edge  indexBase=One  operateOver=Each column  Dimension=1  colComp=on  operation=maximum  roiEnable=off  roiType=Rectangles  roiPortion=Entire ROI  roiOutput=Individual statistics for each ROI  roiFlag=off  accumDataTypeStr=Inherit: Same as product output  accumLastDataTypeStr=Inherit: Same as product output  roundingMode=Floor  overflowMode=off
  Subsystem1 : Subsystem
  Unit Delay : UnitDelay  SampleTime=-1
  Variance : dspstat3/Variance  DialogController=dspDDGCreate  DialogControllerArgs=DataTag4  run=on  reset_popup=Rising edge  directionMode=Each column  dimension=1  treatSBRowAsCol=on  roiEnable=off  roiType=Rectangles  roiPortion=Entire ROI  roiOutput=Individual statistics for each ROI  roiFlag=off  roundingMode=Floor  overflowMode=off
  reset control : Subsystem
  sampled  quantities : Subsystem  TreatAsAtomicUnit=on
  sampled : Outport  OutDataType=sfix(16)  OutScaling=2^0
  1 cycle max p-p : Outport  Port=2  OutDataType=sfix(16)  OutScaling=2^0
  N cycles : Outport  Port=3  OutDataType=sfix(16)  OutScaling=2^0
  Variance1 : Outport  Port=4  OutDataType=sfix(16)  OutScaling=2^0
  wires:
  in/1 -> Gain/1, Variance/1, Difference/1, Subsystem1/1(In1)
  Difference/1 -> Abs/1
  Abs/1 -> Maximum/1
  sample_size/1 -> reset control/1(count)
  reset control/1(Out1) -> Unit Delay/1, sampled  quantities/Trigger, Subsystem1/2(Reset)
  sampled  quantities/1(P-P) -> Gain1/1
  Variance/1 -> sampled  quantities/3(run_var_in)
  sampled  quantities/2(Variance) -> Gain2/1
  Unit Delay/1 -> Variance/2, Maximum/2
  Maximum/1 -> sampled  quantities/4(1_max_in)
  sampled  quantities/3(1_max_out) -> Gain3/1
  Gain/1 -> sampled/1
  Gain1/1 -> N cycles/1
  Gain2/1 -> Variance1/1
  Gain3/1 -> 1 cycle max p-p/1
  Subsystem1/2(Max) -> sampled  quantities/2(Max_in)
  Subsystem1/1(Min) -> sampled  quantities/1(Min_in)

== system fractional_6/Jitter Measurement /sampler & process/Subsystem1 ==
  In1 : Inport  OutDataType=sfix(16)  OutScaling=2^0
  Reset : Inport  Port=2  OutDataType=sfix(16)  OutScaling=2^0
  Maximum1 : dspstat3/Maximum  DialogController=dspDDGCreate  DialogControllerArgs=DataTag2  fcn=Running  reset=Non-zero sample  indexBase=One  operateOver=Each column  Dimension=1  colComp=on  operation=maximum  roiEnable=off  roiType=Rectangles  roiPortion=Entire ROI  roiOutput=Individual statistics for each ROI  roiFlag=off  accumDataTypeStr=Inherit: Same as product output  accumLastDataTypeStr=Inherit: Same as product output  roundingMode=Floor  overflowMode=off
  Minimum : dspstat3/Minimum  DialogController=dspDDGCreate  DialogControllerArgs=DataTag3  fcn=Running  reset=Non-zero sample  indexBase=One  operateOver=Each column  Dimension=1  colComp=on  operation=minimum  roiEnable=off  roiType=Rectangles  roiPortion=Entire ROI  roiOutput=Individual statistics for each ROI  roiFlag=off  roundingMode=Floor  overflowMode=off
  Unit Delay : UnitDelay  SampleTime=-1
  Unit Delay1 : UnitDelay  SampleTime=-1
  Min : Outport  OutDataType=sfix(16)  OutScaling=2^0
  Max : Outport  Port=2  OutDataType=sfix(16)  OutScaling=2^0
  wires:
  Maximum1/1 -> Unit Delay/1
  Minimum/1 -> Unit Delay1/1
  Reset/1 -> Minimum/2, Maximum1/2
  In1/1 -> Minimum/1, Maximum1/1
  Unit Delay/1 -> Max/1
  Unit Delay1/1 -> Min/1

== system fractional_6/Jitter Measurement /sampler & process/reset control ==
  count : Inport  OutDataType=sfix(16)  OutScaling=2^0
  Constant2 : Constant  OutDataType=sfix(16)  OutScaling=2^0
  Fcn4 : Fcn  Expr=u<1
  Math Function : Math  Operator=mod  OutDataType=sfix(16)  OutScaling=2^0  SaturateOnIntegerOverflow=on
  Sum2 : Sum  Inputs=|++  OutDataType=sfix(16)  OutScaling=2^0  SaturateOnIntegerOverflow=on  InputSameDT=on  OutDataTypeStr=Inherit: Same as first input
  Unit Delay1 : UnitDelay  SampleTime=-1
  Out1 : Outport  OutDataType=sfix(16)  OutScaling=2^0
  wires:
  Math Function/1 -> Fcn4/1, Sum2/2
  Unit Delay1/1 -> Math Function/1
  Constant2/1 -> Sum2/1
  Sum2/1 -> Unit Delay1/1
  Fcn4/1 -> Out1/1
  count/1 -> Math Function/2

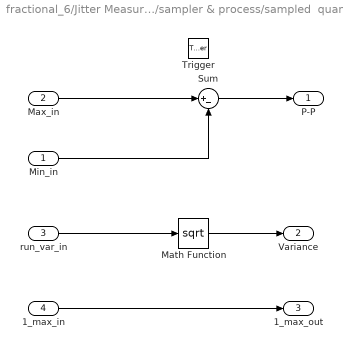
== system fractional_6/Jitter Measurement /sampler & process/sampled  quantities ==
  Min_in : Inport  OutDataType=sfix(16)  OutScaling=2^0
  Max_in : Inport  Port=2  OutDataType=sfix(16)  OutScaling=2^0
  run_var_in : Inport  Port=3  OutDataType=sfix(16)  OutScaling=2^0
  1_max_in : Inport  Port=4  OutDataType=sfix(16)  OutScaling=2^0
  Trigger : TriggerPort
  Math Function : Math  Operator=sqrt  OutDataType=sfix(16)  OutScaling=2^0  SaturateOnIntegerOverflow=on
  Sum : Sum  Inputs=|+-  OutDataType=sfix(16)  OutScaling=2^0  SaturateOnIntegerOverflow=on  InputSameDT=on  OutDataTypeStr=Inherit: Same as first input
  P-P : Outport  OutDataType=sfix(16)  OutScaling=2^0
  Variance : Outport  Port=2  OutDataType=sfix(16)  OutScaling=2^0
  1_max_out : Outport  Port=3  OutDataType=sfix(16)  OutScaling=2^0
  wires:
  Max_in/1 -> Sum/1
  Min_in/1 -> Sum/2
  Sum/1 -> P-P/1
  Math Function/1 -> Variance/1
  run_var_in/1 -> Math Function/1
  1_max_in/1 -> 1_max_out/1
